simulink model "course_design"  (R2024b)
settings: Solver=VariableStepAuto  StartTime=0.0  StopTime=10  RelTol=1e-3
settings Model: Creator=86195  LastModifiedBy=86195

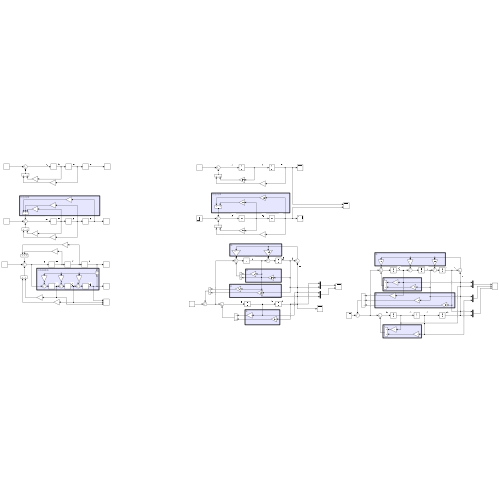
[thumbnail: Simulink's stored preview of the top-level diagram]
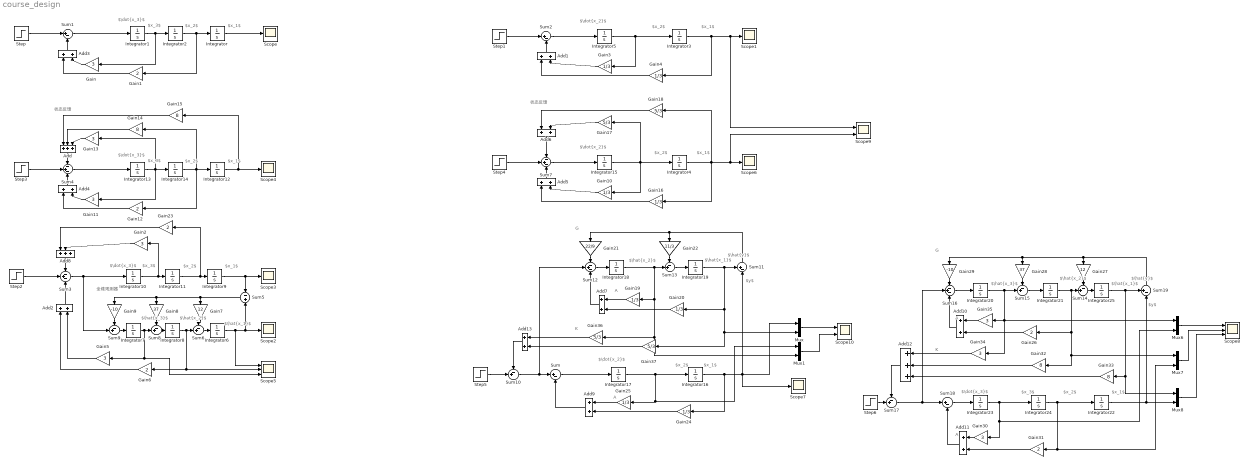
== system course_design ==
  note: $x_2$
  note: $x_3$
  note: $\hat{x_3}$
  note: $x_1$
  note: $\dot{x_3}$
  note: 状态反馈
  note: $\hat{x_1}$
  note: $\hat{x_2}$
  note: $x_1$
  note: 全维观测器
  note: $x_3$
  note: $\dot{x_3}$
  note: $x_1$
  note: $x_3$
  note: $x_2$
  note: $\dot{x_3}$
  note: $x_2$
  note: $x_1$
  note: $\dot{x_2}$
  note: $x_2$
  note: $\dot{x_2}$
  note: $x_1$
  note: $x_2$
  note: 状态反馈
  note: $\dot{x_2}$
  note: $x_1$
  note: $x_2$
  note: $\hat{x_1}$
  note: $\hat{x_2}$
  note: G
  note: A
  note: $y$
  note: G
  note: $\hat{y}$
  note: K
  note: $\hat{x_3}$
  note: $\hat{x_2}$
  note: $\dot{x_3}$
  note: $x_3$
  note: $x_1$
  note: $\hat{x_1}$
  note: A
  note: $x_2$
  note: A
  note: K
  note: A
  note: $\hat{y}$
  note: $y$
  Add : Sum  Inputs=+++
  Add{1..7,9..11,13} (11 alike) : Sum
  Add12 : Sum  Inputs=+++
  Add8 : Sum  Inputs=+++
  Gain{,2,5,11,13,30,34..35} (8 alike) : Gain  Gain=3
  Gain{1,6,12,23,26,31} (6 alike) : Gain  Gain=2
  Gain{3..4,10,16,19..20,24..25} (8 alike) : Gain  Gain=1/3
  Gain{14..15,32..33} (4 alike) : Gain  Gain=8
  Gain{17..18,36..37} (4 alike) : Gain  Gain=5/3
  Gain21 : Gain  Gain=22/9
  Gain22 : Gain  Gain=11/3
  Gain27 : Gain  Gain=12
  Gain28 : Gain  Gain=37
  Gain29 : Gain  Gain=-10
  Gain7 : Gain  Gain=12
  Gain8 : Gain  Gain=37
  Gain9 : Gain  Gain=-10
  Integrator{,1..21,23..25} (25 alike) : Integrator
  Integrator22 : Integrator  InitialCondition=1
  Mux{,1,6..8} (5 alike) : Mux  Inputs=2
  Scope{,1..4,6..7} (7 alike) : Scope
  Scope10 : Scope  NumInputPorts=2
  Scope5 : Scope  NumInputPorts=3
  Scope8 : Scope  NumInputPorts=3
  Scope9 : Scope  NumInputPorts=2
  Step{,1..6} (7 alike) : Step  SampleTime=0
  Sum{,1..2,18} (4 alike) : Sum  Inputs=|+-
  Sum{6,8..10,13..15,17} (8 alike) : Sum  Inputs=-+|
  Sum11 : Sum  Inputs=+-|
  Sum{3..4,7,12,16} (5 alike) : Sum  Inputs=-+-
  Sum19 : Sum  Inputs=+-|
  Sum5 : Sum  Inputs=-|+
  wires:
  Gain8/1 -> Sum8/1
  Step/1 -> Sum1/1
  Gain15/1 -> Add/1
  Gain13/1 -> Add/3
  Gain7/1 -> Sum6/1
  Integrator12/1 -> Gain15/1, Scope4/1
  Gain14/1 -> Add/2
  Gain/1 -> Add3/2
  Integrator/1 -> Scope/1
  Step3/1 -> Sum4/2
  Sum9/1 -> Integrator7/1
  Integrator7/1 -> Gain5/1, Scope5/3, Sum8/2
  Gain1/1 -> Add3/1
  Add/1 -> Sum4/1
  Sum5/1 -> Gain8/1, Gain9/1, Gain7/1
  Add4/1 -> Sum4/3
  Integrator9/1 -> Scope3/1, Sum5/1
  Sum1/1 -> Integrator1/1
  Sum3/1 -> Integrator10/1, Sum9/2
  Integrator1/1 -> Integrator2/1, Gain/1
  Add3/1 -> Sum1/2
  Sum6/1 -> Integrator6/1
  Integrator11/1 -> Gain23/1, Integrator9/1
  Integrator6/1 -> Scope2/1, Sum5/2, Scope5/1
  Integrator8/1 -> Sum6/2, Gain6/1, Scope5/2
  Sum8/1 -> Integrator8/1
  Sum4/1 -> Integrator13/1
  Gain11/1 -> Add4/2
  Gain9/1 -> Sum9/1
  Gain12/1 -> Add4/1
  Integrator14/1 -> Gain14/1, Gain12/1, Integrator12/1
  Integrator2/1 -> Gain1/1, Integrator/1
  Integrator10/1 -> Gain2/1, Integrator11/1
  Gain6/1 -> Add2/1
  Integrator13/1 -> Gain13/1, Gain11/1, Integrator14/1
  Integrator5/1 -> Integrator3/1, Gain3/1
  Gain4/1 -> Add1/1
  Integrator3/1 -> Gain4/1, Scope9/1, Scope1/1
  Gain3/1 -> Add1/2
  Step1/1 -> Sum2/1
  Add1/1 -> Sum2/2
  Sum2/1 -> Integrator5/1
  Sum7/1 -> Integrator15/1
  Gain16/1 -> Add5/1
  Integrator15/1 -> Gain17/1, Integrator4/1, Gain10/1
  Gain10/1 -> Add5/2
  Integrator4/1 -> Gain18/1, Gain16/1, Scope9/2, Scope6/1
  Step4/1 -> Sum7/2
  Add5/1 -> Sum7/3
  Add6/1 -> Sum7/1
  Gain17/1 -> Add6/2
  Gain18/1 -> Add6/1
  Sum10/1 -> Sum/1, Sum12/2
  Integrator17/1 -> Integrator16/1, Mux1/1, Gain25/1
  Integrator16/1 -> Mux/1, Scope7/1, Sum11/2, Gain24/1
  Gain5/1 -> Add2/2
  Step2/1 -> Sum3/2
  Add2/1 -> Sum3/3
  Add8/1 -> Sum3/1
  Gain2/1 -> Add8/2
  Gain23/1 -> Add8/1
  Step5/1 -> Sum10/2
  Add13/1 -> Sum10/1
  Gain22/1 -> Sum13/1
  Gain21/1 -> Sum12/1
  Sum12/1 -> Integrator18/1
  Sum13/1 -> Integrator19/1
  Sum11/1 -> Gain22/1, Gain21/1
  Add11/1 -> Sum18/2
  Mux6/1 -> Scope8/1
  Mux8/1 -> Scope8/3
  Add10/1 -> Sum16/3
  Gain28/1 -> Sum15/1
  Gain30/1 -> Add11/1
  Gain29/1 -> Sum16/1
  Sum19/1 -> Gain29/1, Gain28/1, Gain27/1
  Sum17/1 -> Sum18/1, Sum16/2
  Sum16/1 -> Integrator20/1
  Integrator20/1 -> Sum15/2, Mux6/1, Gain35/1, Gain34/1
  Integrator21/1 -> Sum14/2, Gain32/1, Mux7/1, Gain26/1
  Sum15/1 -> Integrator21/1
  Sum14/1 -> Integrator25/1
  Add12/1 -> Sum17/1
  Mux7/1 -> Scope8/2
  Gain31/1 -> Add11/2
  Gain34/1 -> Add12/1
  Integrator25/1 -> Sum19/1, Mux8/1, Gain33/1
  Step6/1 -> Sum17/2
  Gain35/1 -> Add10/1
  Integrator23/1 -> Integrator24/1, Gain30/1, Mux6/2
  Gain32/1 -> Add12/2
  Gain33/1 -> Add12/3
  Integrator24/1 -> Integrator22/1, Gain31/1, Mux7/2
  Sum18/1 -> Integrator23/1
  Gain27/1 -> Sum14/1
  Gain26/1 -> Add10/2
  Integrator22/1 -> Mux8/2, Sum19/2
  Gain19/1 -> Add7/1
  Gain20/1 -> Add7/2
  Add9/1 -> Sum/2
  Add7/1 -> Sum12/3
  Integrator19/1 -> Sum11/1, Mux/2, Gain37/1, Gain20/1
  Integrator18/1 -> Sum13/2, Mux1/2, Gain36/1, Gain19/1
  Gain37/1 -> Add13/2
  Gain36/1 -> Add13/1
  Gain25/1 -> Add9/1
  Gain24/1 -> Add9/2
  Sum/1 -> Integrator17/1
  Mux/1 -> Scope10/1
  Mux1/1 -> Scope10/2
